simulink model "Model"  (Simulink 8.2)
settings: Solver=ode23  StartTime=-1  StopTime=Tsim  RelTol=1e-5  AbsTol=1e-6
values from neighbouring files (symbols this model uses):
  deltainit = asin(pm / pemax)    [Ulazni_podaci.m]
  PD = 0.00    (= 0)    [Ulazni_podaci.m]
  peimax = 1.3750    (= 1.375)    [Ulazni_podaci.m]
  pekmax = 0.9275    [Ulazni_podaci.m]
  pemax = 1.6090    (= 1.609)    [Ulazni_podaci.m]
  pm = 0.9000    (= 0.9)    [Ulazni_podaci.m]
  Ti = 5    [Ulazni_podaci.m]
  wnom = 2*pi*f    (= 314.159265359)    [Ulazni_podaci.m]
libraries: simulink x2
settings Model: Creator=BOJAN  LastModifiedBy=Bojan
settings SolverCC: ShapePreserveControl=EnableAll
settings DataIOCC: SignalLoggingSaveFormat=Dataset
settings OptimizationCC: ExpressionDepthLimit=128
settings DebuggingCC: FcnCallInpInsideContextMsg=EnableAllAsError  StateNameClashWarn=none
settings GRTTargetCC: CombineOutputUpdateFcns=on  GRTInterface=off

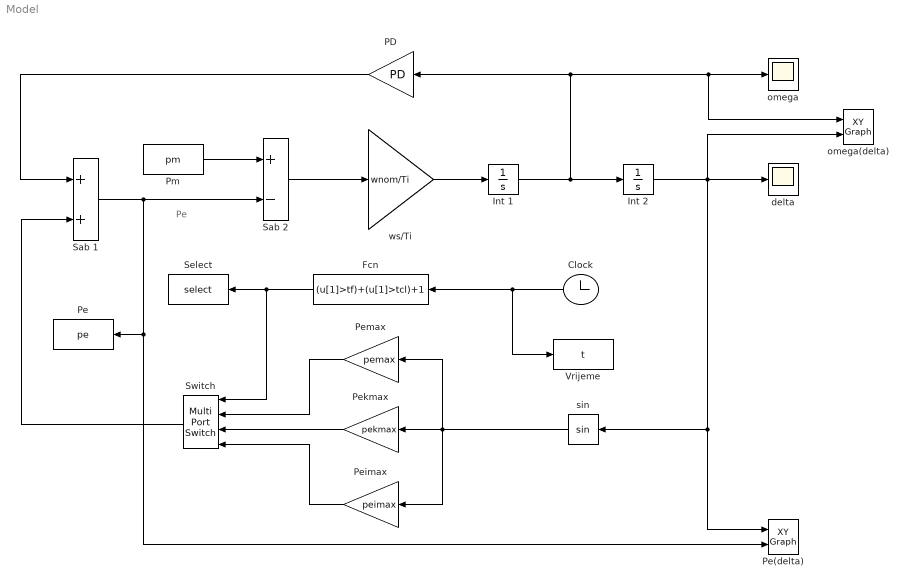
== system Model ==
  note: Pe
  " Sab 1    " : Sum
  Clock : Clock
  Fcn : Fcn  Expr=(u[1]>tf)+(u[1]>tcl)+1
  Int 1 : Integrator
  Int 2 : Integrator  InitialCondition=deltainit
  PD : Gain  Gain=PD
  Pe : ToWorkspace  VariableName=pe  SampleTime=-1
  Pe(delta) : simulink/Sinks/XY Graph  xmin=0  xmax=pi  ymin=0  ymax=2.5  st=-1
  Peimax : Gain  Gain=peimax
  Pekmax : Gain  Gain=pekmax
  Pemax : Gain  Gain=pemax
  Pm : Constant  Value=pm
  Sab 2 : Sum  Inputs=+-
  Select : ToWorkspace  VariableName=select  SampleTime=-1
  Switch : MultiPortSwitch
  Vrijeme : ToWorkspace  VariableName=t  SampleTime=-1
  delta : Scope
      settings: YMin=2500  YMax=11500  SaveName=delta
  omega : Scope
      settings: SaveName=omega
  omega(delta) : simulink/Sinks/XY Graph  xmin=-15  xmax=15  ymin=-5  ymax=5  st=-1
  sin : Trigonometry
  "ws/Ti  " : Gain  Gain=wnom/Ti
  wires:
  Pm/1 -> Sab 2/1
  Sab 2/1 -> "ws/Ti  "/1
  "ws/Ti  "/1 -> Int 1/1
  Int 1/1 -> omega(delta)/1, omega/1, PD/1, Int 2/1
  Int 2/1 -> omega(delta)/2, Pe(delta)/1, sin/1, delta/1
  " Sab 1    "/1 -> Pe/1, Pe(delta)/2, Sab 2/2
  PD/1 -> " Sab 1    "/1
  Fcn/1 -> Select/1, Switch/1
  Clock/1 -> Fcn/1, Vrijeme/1
  sin/1 -> Peimax/1, Pemax/1, Pekmax/1
  Pekmax/1 -> Switch/3
  Pemax/1 -> Switch/2
  Peimax/1 -> Switch/4
  Switch/1 -> " Sab 1    "/2
